simulink model "chap1_8"  (R2016a)
settings: Solver=ode45  StartTime=0.0  StopTime=2  RelTol=1e-3
settings Model: Creator=admin  LastModifiedBy=admin

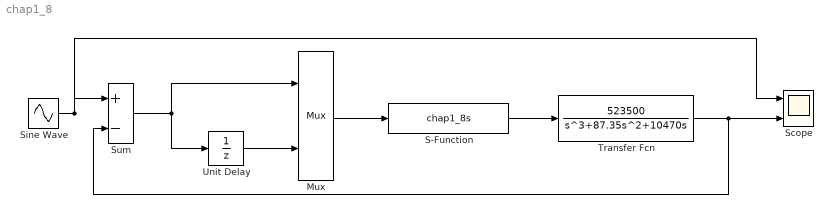
== system chap1_8 ==
  Mux : Mux  Inputs=2
  S-Function : S-Function  FunctionName=chap1_8s  SFunctionDeploymentMode=off  EnableBusSupport=off
  Scope : Scope  NumInputPorts=2
  Sine Wave : Sin  Frequency=2*pi  SampleTime=0
  Sum : Sum  Inputs=|+-
  Transfer Fcn : TransferFcn  Numerator=[523500]  Denominator=[1 87.35 10470 0]
  Unit Delay : UnitDelay  SampleTime=0.001
  wires:
  Sine Wave/1 -> Scope/1, Sum/1
  Unit Delay/1 -> Mux/2
  Sum/1 -> Unit Delay/1, Mux/1
  S-Function/1 -> Transfer Fcn/1
  Mux/1 -> S-Function/1
  Transfer Fcn/1 -> Sum/2, Scope/2
